simulink model "ACS_2_my"  (R2017b)
settings: Solver=ode45  StartTime=0.0  StopTime=10  RelTol=1e-3  EnableMultiTasking=on
settings Model: Creator=Vano  LastModifiedBy=Ruslan
settings DataIOCC: LimitDataPoints=on  SaveFormat=Array  SignalLoggingSaveFormat=ModelDataLogs
settings OptimizationCC: ExpressionDepthLimit=2147483647  LifeSpan=inf
settings DebuggingCC: UnderspecifiedInitializationDetection=Classic  MergeDetectMultiDrivingBlocksExec=none  SolverPrmCheckMsg=warning  FcnCallInpInsideContextMsg=warning  StateNameClashWarn=warning  SFUnexpectedBacktrackingDiag=warning  SFNoUnconditionalDefaultTransitionDiag=warning  SFExecutionAtInitializationDiag=none
settings HardwareCC: ProdBitPerPointer=32  ProdBitPerSizeT=32  ProdBitPerPtrDiffT=32  ProdLargestAtomicFloat=None  ProdIntDivRoundTo=Undefined  ProdEndianess=Unspecified  ProdWordSize=32  ProdHWDeviceType=32-bit Generic
settings ModelReferenceCC: PropagateSignalLabelsOutOfModel=off
settings CodeAppCC: StateflowObjectComments=on
settings GRTTargetCC: TargetLangStandard=C89/C90 (ANSI)  CombineOutputUpdateFcns=off  GRTInterface=on
settings ConfigComp: CovMetricSettings=dw  CovHtmlReporting=on  CovSaveCumulativeToWorkspaceVar=on  CovSaveSingleToWorkspaceVar=on  CovExternalEMLEnable=off

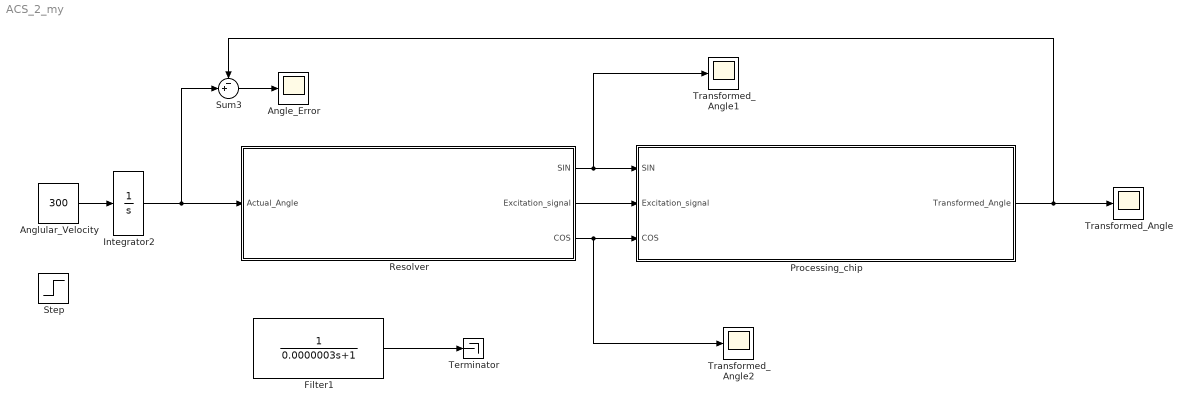
== system ACS_2_my ==
  Angle_Error : Scope
  Anglular_Velocity : Constant  Value=300
  Filter1 : TransferFcn  Denominator=[0.0000003 1]
  Integrator2 : Integrator
  Processing_chip : Subsystem
  Resolver : Subsystem
  Step : Step  Time=0  SampleTime=0
  Sum3 : Sum  Inputs=-+|
  Terminator : Terminator
  Transformed_Angle : Scope
  Transformed_Angle1 : Scope
  Transformed_Angle2 : Scope
  wires:
  Sum3/1 -> Angle_Error/1
  Filter1/1 -> Terminator/1
  Processing_chip/1(Transformed_Angle) -> Transformed_Angle/1, Sum3/1
  Resolver/1(SIN) -> Processing_chip/1(SIN), Transformed_Angle1/1
  Resolver/3(COS) -> Processing_chip/3(COS), Transformed_Angle2/1
  Resolver/2(Excitation_signal) -> Processing_chip/2(Excitation_signal)
  Anglular_Velocity/1 -> Integrator2/1
  Integrator2/1 -> Resolver/1(Actual_Angle), Sum3/2

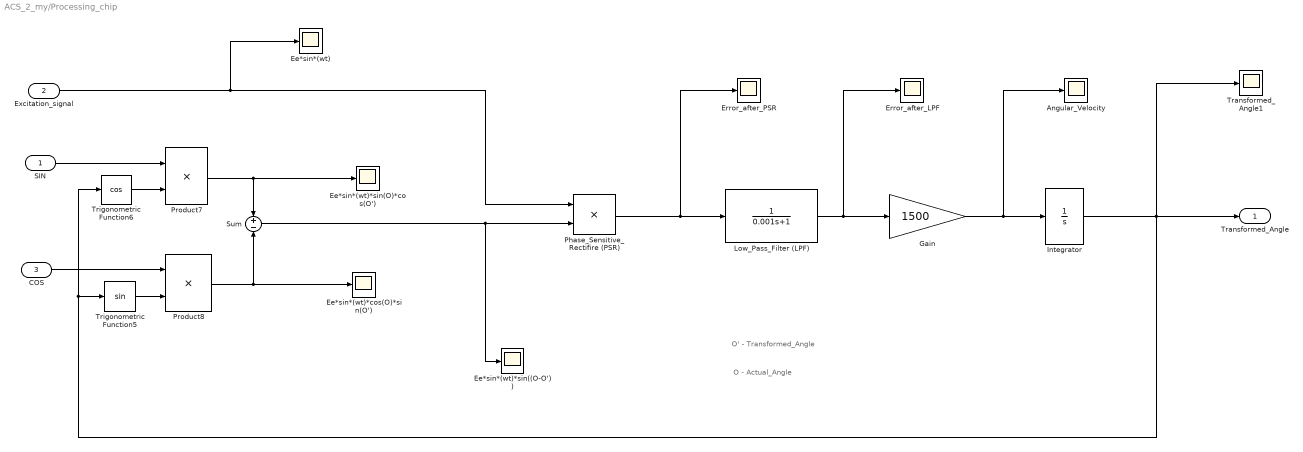
== system ACS_2_my/Processing_chip ==
  note: O' - Transformed_Angle
  note: O - Actual_Angle
  SIN : Inport
  Excitation_signal : Inport  Port=2
  COS : Inport  Port=3
  Angular_Velocity : Scope
  Ee*sin*(wt) : Scope
  Ee*sin*(wt)*cos(O)*sin(O') : Scope
  Ee*sin*(wt)*sin((O-O')) : Scope
  Ee*sin*(wt)*sin(O)*cos(O') : Scope
  Error_after_LPF : Scope
  Error_after_PSR : Scope
  Gain : Gain  Gain=1500
  Integrator : Integrator
  Low_Pass_Filter (LPF) : TransferFcn  Denominator=[0.001 1]
  Phase_Sensitive_Rectifire (PSR) : Product  RndMeth=Zero
  Product7 : Product  RndMeth=Zero
  Product8 : Product  RndMeth=Zero
  Sum : Sum  Inputs=+-
  Transformed_Angle1 : Scope
  Trigonometric Function5 : Trigonometry
  Trigonometric Function6 : Trigonometry  Operator=cos
  Transformed_Angle : Outport
  wires:
  Trigonometric Function6/1 -> Product7/2
  Trigonometric Function5/1 -> Product8/2
  Product7/1 -> Sum/1, Ee*sin*(wt)*sin(O)*cos(O')/1
  Product8/1 -> Sum/2, Ee*sin*(wt)*cos(O)*sin(O')/1
  SIN/1 -> Product7/1
  COS/1 -> Product8/1
  Excitation_signal/1 -> Phase_Sensitive_Rectifire (PSR)/1, Ee*sin*(wt)/1
  Phase_Sensitive_Rectifire (PSR)/1 -> Low_Pass_Filter (LPF)/1, Error_after_PSR/1
  Sum/1 -> Phase_Sensitive_Rectifire (PSR)/2, Ee*sin*(wt)*sin((O-O'))/1
  Low_Pass_Filter (LPF)/1 -> Gain/1, Error_after_LPF/1
  Gain/1 -> Integrator/1, Angular_Velocity/1
  Integrator/1 -> Transformed_Angle/1, Trigonometric Function6/1, Trigonometric Function5/1, Transformed_Angle1/1

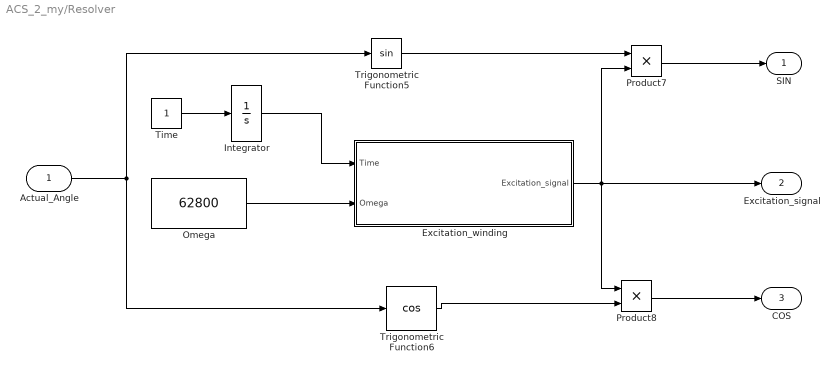
== system ACS_2_my/Resolver ==
  Actual_Angle : Inport
  Excitation_winding : Subsystem
  Integrator : Integrator
  Omega : Constant  Value=62800
  Product7 : Product  RndMeth=Zero
  Product8 : Product  RndMeth=Zero
  Time : Constant
  Trigonometric Function5 : Trigonometry
  Trigonometric Function6 : Trigonometry  Operator=cos
  SIN : Outport
  Excitation_signal : Outport  Port=2
  COS : Outport  Port=3
  wires:
  Time/1 -> Integrator/1
  Integrator/1 -> Excitation_winding/1(Time)
  Omega/1 -> Excitation_winding/2(Omega)
  Actual_Angle/1 -> Trigonometric Function6/1, Trigonometric Function5/1
  Trigonometric Function6/1 -> Product8/2
  Trigonometric Function5/1 -> Product7/1
  Excitation_winding/1(Excitation_signal) -> Product7/2, Product8/1, Excitation_signal/1
  Product7/1 -> SIN/1
  Product8/1 -> COS/1

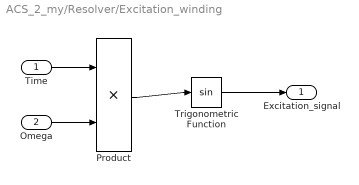
== system ACS_2_my/Resolver/Excitation_winding ==
  Time : Inport
  Omega : Inport  Port=2
  Product : Product  RndMeth=Zero
  Trigonometric Function : Trigonometry
  Excitation_signal : Outport
  wires:
  Omega/1 -> Product/2
  Trigonometric Function/1 -> Excitation_signal/1
  Time/1 -> Product/1
  Product/1 -> Trigonometric Function/1
